simulink model "fz8_11"  (R2014a)
settings: Solver=ode45  StartTime=0.0  StopTime=10.0  RelTol=1e-3
values from neighbouring files (symbols this model uses):
  BitRate = 100000    [eg8_11.m]
  Lc = 7    [eg8_11.m]
libraries: commcnvcod2 x3, commdigbbndpm3 x2, commsink2 x2, commchan3 x1, commrandsrc2 x1
settings Model: Creator=tzb  LastModifiedBy=tzb

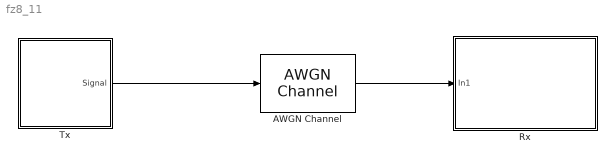
== system fz8_11 ==
  AWGN Channel : commchan3/AWGN Channel  InputProcessing=Columns as channels (frame based)  seed=67  noiseMode="Signal to noise ratio  (Eb/No)"  EbNodB=SNR  EsNodB=10  SNRdB=10  bitsPerSym=1  Ps=1  Tsym=1/BitRate  variance=1
  "Rx " : Subsystem
  Tx : Subsystem
  wires:
  Tx/1(Signal) -> AWGN Channel/1
  AWGN Channel/1 -> "Rx "/1(In1)

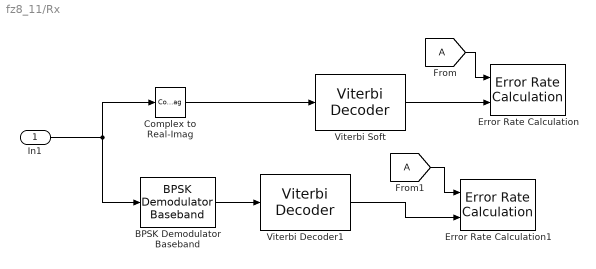
== system fz8_11/Rx  ==
  In1 : Inport
  BPSK Demodulator Baseband : commdigbbndpm3/BPSK Demodulator Baseband  Ph=0  DecType=Hard decision  VarSource=Dialog  Variance=1  outDtype=Inherit via internal rule  derotateFactorWordLen=16
  Complex to Real-Imag : ComplexToRealImag  Output=Real
  Error Rate Calculation : commsink2/Error Rate Calculation  N=0  st_delay=6*Lc  cp_mode=Entire frame  subframe=[]  PMode=Workspace  WsName=BER1  RsMode2=off  stop=off  numErr=100  maxBits=1e6
  Error Rate Calculation1 : commsink2/Error Rate Calculation  N=0  st_delay=6*Lc  cp_mode=Entire frame  subframe=[]  PMode=Workspace  WsName=BER2  RsMode2=off  stop=off  numErr=100  maxBits=1e6
  Viterbi Decoder1 : commcnvcod2/Viterbi Decoder  trellis=poly2trellis(Lc, [171 133])  isPunctured=off  punctureVector=[1; 1; 0; 1; 0; 1]  erasures=off  dectype=Hard decision  runSigValErrCheck=off  nsdecb=4  smWordLength=16  tbdepth=6*Lc  opmode=Continuous  reset=off  outDataType=Inherit via internal rule  delayedResetAction=off
  Viterbi Soft : commcnvcod2/Viterbi Decoder  trellis=poly2trellis(Lc, [171 133])  isPunctured=off  punctureVector=[1; 1; 0; 1; 0; 1]  erasures=off  dectype=Soft decision  runSigValErrCheck=off  nsdecb=4  smWordLength=16  tbdepth=6*Lc  opmode=Continuous  reset=off  outDataType=Inherit via internal rule  delayedResetAction=off
  wires:
  In1/1 -> Complex to Real-Imag/1, BPSK Demodulator Baseband/1
  Complex to Real-Imag/1 -> Viterbi Soft/1
  [A] -> Error Rate Calculation/1
  Viterbi Soft/1 -> Error Rate Calculation/2
  [A] -> Error Rate Calculation1/1
  Viterbi Decoder1/1 -> Error Rate Calculation1/2
  BPSK Demodulator Baseband/1 -> Viterbi Decoder1/1

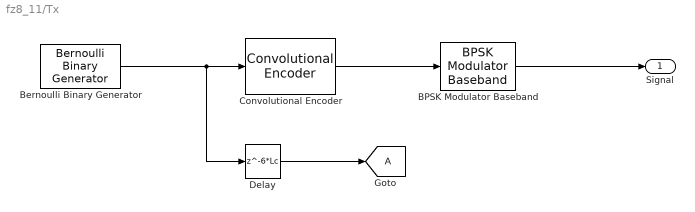
== system fz8_11/Tx ==
  BPSK Modulator Baseband : commdigbbndpm3/BPSK Modulator Baseband  Ph=0  outDtype=double  outWordLen=16  outUDDataType=sfix(16)  outFracLenMode=Best precision  outFracLen=15
  Bernoulli Binary Generator : commrandsrc2/Bernoulli Binary Generator  P=0.5  seed=61  Ts=1/BitRate  frameBased=on  sampPerFrame=BitRate  orient=off  outDataType=double
  Convolutional Encoder : commcnvcod2/Convolutional Encoder  trellis=poly2trellis(Lc, [171 133])  opMode=Continuous  DelayedResetAction=off  hasIniStPort=off  hasFinStPort=off  usePuncVector=off  punctureVector=[1; 1; 0; 1; 0; 1]  reset=Unused parameter value
  Delay : Delay  DelayLength=6*Lc  InitialCondition=0  InputProcessing=Inherited
  Signal : Outport
  tag scope: A=global
  wires:
  BPSK Modulator Baseband/1 -> Signal/1
  Convolutional Encoder/1 -> BPSK Modulator Baseband/1
  Bernoulli Binary Generator/1 -> Delay/1, Convolutional Encoder/1
  Delay/1 -> [A]
